simulink library "INP_UNSP_Prep"  (R2024b)
settings: Solver=VariableStepAuto  StartTime=0.0  StopTime=10.0  RelTol=1e-3
undefined symbols (not defined in the file): INP_c_TiSample_s, INP_p_TiTau_s, INP_UNSP_p_AccUnspOfsFrLe_mps2, INP_UNSP_p_AccUnspOfsFrRi_mps2, INP_UNSP_p_AccUnspOfsReLe_mps2, INP_UNSP_p_AccUnspOfsReRi_mps2, INP_UNSP_p_AccUnspScaFrLe_na, INP_UNSP_p_AccUnspScaFrRi_na, INP_UNSP_p_AccUnspScaReLe_na, INP_UNSP_p_AccUnspScaReRi_na
libraries: VUT_lib x4
settings Model: Creator=blatak  LastModifiedBy=blatak

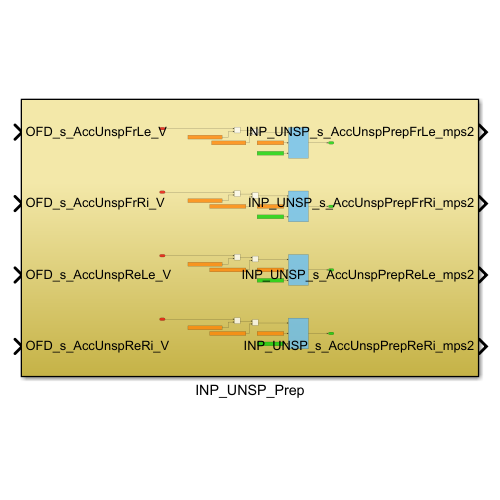
[thumbnail: Simulink's stored preview of the top-level diagram]
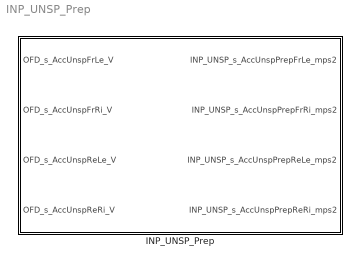
== system INP_UNSP_Prep ==
  INP_UNSP_Prep : Subsystem

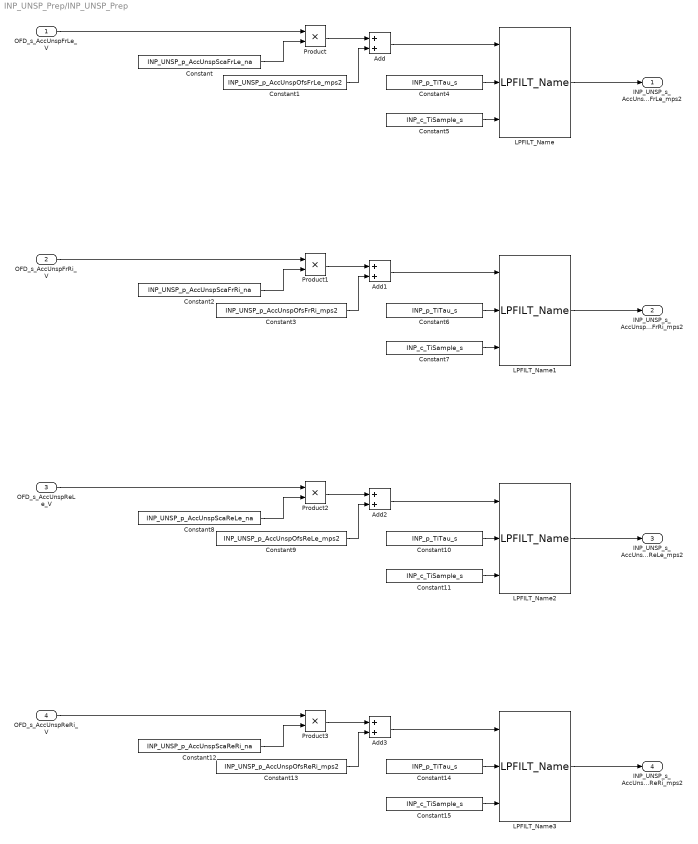
== system INP_UNSP_Prep/INP_UNSP_Prep ==
  OFD_s_AccUnspFrLe_V : Inport
  OFD_s_AccUnspFrRi_V : Inport  Port=2
  OFD_s_AccUnspReLe_V : Inport  Port=3
  OFD_s_AccUnspReRi_V : Inport  Port=4
  Add{,1..3} (4 alike) : Sum
  Constant : Constant  Description=Scaling coefficient to recalculate the electric quantity to the physical one - longitudinal acceleration  Value=INP_UNSP_p_AccUnspScaFrLe_na
  Constant1 : Constant  Description=Offset to recalculate the electric quantity to the physical one - longitudinal acceleration  Value=INP_UNSP_p_AccUnspOfsFrLe_mps2
  Constant{4,6,10,14} (4 alike) : Constant  Value=INP_p_TiTau_s
  Constant{5,7,11,15} (4 alike) : Constant  Value=INP_c_TiSample_s
  Constant12 : Constant  Description=Scaling coefficient to recalculate the electric quantity to the physical one - longitudinal acceleration  Value=INP_UNSP_p_AccUnspScaReRi_na
  Constant13 : Constant  Description=Offset to recalculate the electric quantity to the physical one - longitudinal acceleration  Value=INP_UNSP_p_AccUnspOfsReRi_mps2
  Constant2 : Constant  Description=Scaling coefficient to recalculate the electric quantity to the physical one - longitudinal acceleration  Value=INP_UNSP_p_AccUnspScaFrRi_na
  Constant3 : Constant  Description=Offset to recalculate the electric quantity to the physical one - longitudinal acceleration  Value=INP_UNSP_p_AccUnspOfsFrRi_mps2
  Constant8 : Constant  Description=Scaling coefficient to recalculate the electric quantity to the physical one - longitudinal acceleration  Value=INP_UNSP_p_AccUnspScaReLe_na
  Constant9 : Constant  Description=Offset to recalculate the electric quantity to the physical one - longitudinal acceleration  Value=INP_UNSP_p_AccUnspOfsReLe_mps2
  LPFILT_Name{,1..3} (4 alike) : VUT_lib/LPFILT_Name  SystemSampleTime=-1  VariantActivationTime=update diagram  AllowFlexibleInterface=on  Latency=0  AutoFrameSizeCalculation=off
  Product{,1..3} (4 alike) : Product
  INP_UNSP_s_AccUnspPrepFrLe_mps2 : Outport
  INP_UNSP_s_AccUnspPrepFrRi_mps2 : Outport  Port=2
  INP_UNSP_s_AccUnspPrepReLe_mps2 : Outport  Port=3
  INP_UNSP_s_AccUnspPrepReRi_mps2 : Outport  Port=4
  wires:
  LPFILT_Name/1 -> INP_UNSP_s_AccUnspPrepFrLe_mps2/1
  OFD_s_AccUnspFrRi_V/1 -> Product1/1
  Add/1 -> LPFILT_Name/1
  Constant5/1 -> LPFILT_Name/3
  LPFILT_Name3/1 -> INP_UNSP_s_AccUnspPrepReRi_mps2/1
  Constant11/1 -> LPFILT_Name2/3
  Constant13/1 -> Add3/2
  Constant3/1 -> Add1/2
  Constant7/1 -> LPFILT_Name1/3
  Product1/1 -> Add1/1
  Constant12/1 -> Product3/2
  Constant2/1 -> Product1/2
  Constant8/1 -> Product2/2
  Add1/1 -> LPFILT_Name1/1
  OFD_s_AccUnspFrLe_V/1 -> Product/1
  Product/1 -> Add/1
  Constant14/1 -> LPFILT_Name3/2
  Constant6/1 -> LPFILT_Name1/2
  OFD_s_AccUnspReLe_V/1 -> Product2/1
  Constant/1 -> Product/2
  Product3/1 -> Add3/1
  Constant4/1 -> LPFILT_Name/2
  Constant9/1 -> Add2/2
  Add3/1 -> LPFILT_Name3/1
  Product2/1 -> Add2/1
  Constant15/1 -> LPFILT_Name3/3
  Constant10/1 -> LPFILT_Name2/2
  OFD_s_AccUnspReRi_V/1 -> Product3/1
  LPFILT_Name2/1 -> INP_UNSP_s_AccUnspPrepReLe_mps2/1
  Constant1/1 -> Add/2
  LPFILT_Name1/1 -> INP_UNSP_s_AccUnspPrepFrRi_mps2/1
  Add2/1 -> LPFILT_Name2/1
